simulink library "mech_fceng_vrlib"  (Simulink 7.1)
libraries: mblibv1 x4, vrlib x1
settings Model: Creator=arnav  LastModifiedBy=batserve

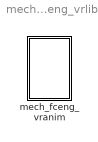
== system mech_fceng_vrlib ==
  mech_fceng_vranim : Subsystem

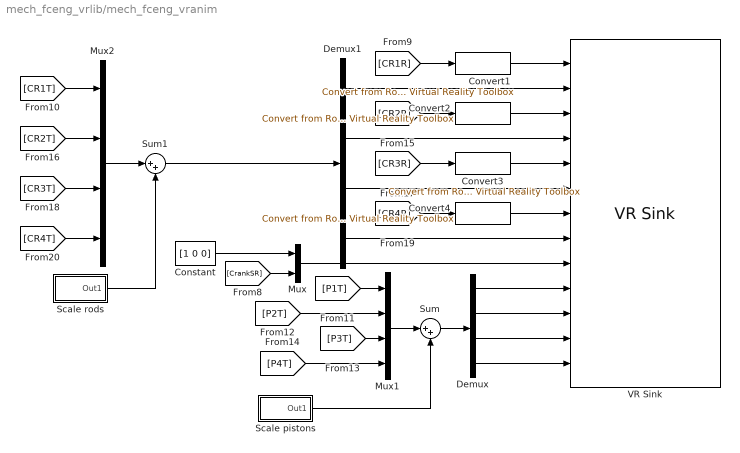
== system mech_fceng_vrlib/mech_fceng_vranim ==
  Constant : Constant  Value=[1 0 0]  OutDataType=sfix(16)  OutScaling=2^0
  Convert{1..4} (4 alike) : mblibv1/Utilities/Convert from Rotation Matrix to Virtual Reality Toolbox  Tag=Pose2VR
  Demux : Demux
  Demux1 : Demux
  Mux : Mux  Inputs=2
  Mux1 : Mux
  Mux2 : Mux
  Scale pistons : Subsystem
  Scale rods : Subsystem
  Sum : Sum  Inputs=|++  OutDataType=sfix(16)  OutScaling=2^0  SaturateOnIntegerOverflow=on  InputSameDT=on  OutDataTypeStr=Inherit: Same as first input
  Sum1 : Sum  Inputs=|++  OutDataType=sfix(16)  OutScaling=2^0  SaturateOnIntegerOverflow=on  InputSameDT=on  OutDataTypeStr=Inherit: Same as first input
  VR Sink : vrlib/VR Sink  SampleTime=0.01  ViewEnable=on  RemoteChange=off  RemoteView=on  FieldsWritten=ConnRod1.rotation#ConnRod1.translation#ConnRod2.rotation#ConnRod2.translation#ConnRod3.rotation#ConnRod3.translation#ConnRod4.rotation#ConnRod4.translation#CrankShaft.rotation#Piston1.translation#Piston2.translation#Piston3.translation#Piston4.translation  WorldFileName=mech_fourcylniceng.wrl  WorldDescription=Four Cylinder Engine Demo  AutoView=off  VideoDimensions=[]  FigureProperties={'Position', 'Name', 'Viewpoint', 'CameraBound', 'CameraDirection', 'CameraPosition', 'CameraUpVector', 'ZoomFactor', 'Antialiasing', 'Headlight', 'Lighting', 'PanelMode', 'Textures', 'Transparency', 'Wireframe', 'DeleteFcn', ; }
  wires:
  [CR2R] -> Convert2/1
  [CR1R] -> Convert1/1
  Convert1/1 -> VR Sink/1
  Convert2/1 -> VR Sink/3
  [CR3R] -> Convert3/1
  Convert3/1 -> VR Sink/5
  [CR4R] -> Convert4/1
  Convert4/1 -> VR Sink/7
  Mux/1 -> VR Sink/9
  Constant/1 -> Mux/1
  [CrankSR] -> Mux/2
  [P1T] -> Mux1/1
  [P2T] -> Mux1/2
  [P3T] -> Mux1/3
  [P4T] -> Mux1/4
  Mux1/1 -> Sum/1
  Scale pistons/1(Out1) -> Sum/2
  Sum/1 -> Demux/1
  Demux/1 -> VR Sink/10
  Demux/2 -> VR Sink/11
  Demux/3 -> VR Sink/12
  Demux/4 -> VR Sink/13
  [CR1T] -> Mux2/1
  [CR2T] -> Mux2/2
  [CR3T] -> Mux2/3
  [CR4T] -> Mux2/4
  Mux2/1 -> Sum1/1
  Scale rods/1(Out1) -> Sum1/2
  Demux1/1 -> VR Sink/2
  Demux1/2 -> VR Sink/4
  Demux1/3 -> VR Sink/6
  Demux1/4 -> VR Sink/8
  Sum1/1 -> Demux1/1

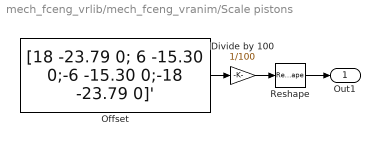
== system mech_fceng_vrlib/mech_fceng_vranim/Scale pistons ==
  Divide by 100 : Gain  Gain=1/100  ParameterDataType=sfix(16)  ParameterScaling=2^0  OutDataType=sfix(16)  OutScaling=2^0  SaturateOnIntegerOverflow=on  OutDataTypeStr=Inherit: Same as input  ParamDataTypeStr=Inherit: Same as input
  Offset : Constant  Value=[18 -23.79 0; 6 -15.30 0;-6 -15.30 0;-18 -23.79 0]'  OutDataType=sfix(16)  OutScaling=2^0
  Reshape : Reshape
  Out1 : Outport
  wires:
  Offset/1 -> Divide by 100/1
  Divide by 100/1 -> Reshape/1
  Reshape/1 -> Out1/1

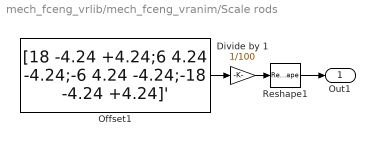
== system mech_fceng_vrlib/mech_fceng_vranim/Scale rods ==
  Divide by 1 : Gain  Gain=1/100  ParameterDataType=sfix(16)  ParameterScaling=2^0  OutDataType=sfix(16)  OutScaling=2^0  SaturateOnIntegerOverflow=on  OutDataTypeStr=Inherit: Same as input  ParamDataTypeStr=Inherit: Same as input
  Offset1 : Constant  Value=[18 -4.24 +4.24;6 4.24 -4.24;-6 4.24 -4.24;-18 -4.24 +4.24]'  OutDataType=sfix(16)  OutScaling=2^0
  Reshape1 : Reshape
  Out1 : Outport
  wires:
  Offset1/1 -> Divide by 1/1
  Divide by 1/1 -> Reshape1/1
  Reshape1/1 -> Out1/1
